simulink model "step9_power_5"  (R2025a)
settings: Solver=ode45  StartTime=0.0  StopTime=20  MaxStep=0.01  RelTol=1e-3
undefined symbols (not defined in the file or in its folder): A, B, F, K, R
libraries: SignalEditorBlockLib x1
settings Model: Creator=O M E N  LastModifiedBy=O M E N

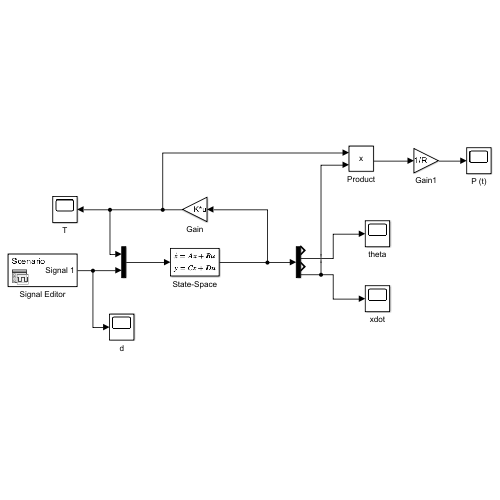
[thumbnail: Simulink's stored preview of the top-level diagram]
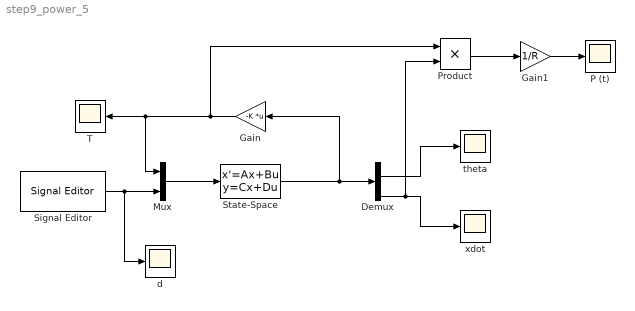
== system step9_power_5 ==
  Demux : Demux
  Gain : Gain  Gain=-K  Multiplication=Matrix(K*u)
  Gain1 : Gain  Gain=1/R
  Mux : Mux  Inputs=2
  P (t) : Scope
      settings: Title=Mechanical power P(t)  ActiveDisplayYMinimum=-695.23617050580935  ActiveDisplayYMaximum=874.09344567927542  YLabel="P  (W)"  DataLoggingVariableName=ScopeData4
  Product : Product
  Signal Editor : SignalEditorBlockLib/Signal Editor  FileName=d_trapezoid.mat  ActiveScenario=Scenario  ActiveSignal=Signal 1  IsBus=off  OutputBusObjectStr=Bus: BusObject  SampleTime=0  ZeroCross=off  OutputAfterFinalValue=Setting to zero  Unit=inherit  PreserveSignalName=on  ApplySigPropsToAllScenarios=on  ApplySigPropsToAllSignals=off  SignalPropertySource=Dialog parameters
  State-Space : StateSpace  A=A  B=[B F]  C=eye(4)  D=zeros(4,2)  InitialCondition=[0; 0; 0; 0]
  T : Scope
      settings: Title=Control torque T(t)  ActiveDisplayYMinimum=-165.7994783180452  ActiveDisplayYMaximum=174.62847831801764  YLabel="T  (N·m)"  DataLoggingVariableName=ScopeData2
  d : Scope
      settings: Title=Disturbance d(t)  ActiveDisplayYMinimum=-0.0012499999999999998  ActiveDisplayYMaximum=0.01125  YLabel="d  (m)"  DataLoggingVariableName=ScopeData3
  theta : Scope
      settings: Title=Tilt angle θ(t)  ActiveDisplayYMinimum=-0.12793257816269588  ActiveDisplayYMaximum=0.1279325781627938  YLabel="θ  (rad)"
  xdot : Scope
      settings: Title=Vehicle speed ẋ(t)  ActiveDisplayYMinimum=-0.55198882805061267  ActiveDisplayYMaximum=3.0745602566061336  YLabel="ẋ  (m/s)"
  wires:
  Mux/1 -> State-Space/1
  State-Space/1 -> Gain/1, Demux/1
  Demux/2 -> theta/1
  Demux/4 -> Product/2, xdot/1
  Gain/1 -> Product/1, T/1, Mux/1
  Signal Editor/1 -> d/1, Mux/2
  Product/1 -> Gain1/1
  Gain1/1 -> P (t)/1
